simulink model "positionModeTest"  (R2022a)
settings: Solver=FixedStepAuto  StartTime=0.0  StopTime=10  FixedStep=sampleTime  RelTol=1e-3
values from neighbouring files (symbols this model uses):
  coulombTorqueNegative = theta(4)/theta(2)    [LeastSquare.m]    (also in leastSquare.m; velRide.m = resultFitNeg(2); velocityRide.m = resultFitNeg(2))
  coulombTorquePositive = theta(3)/theta(2)    [LeastSquare.m]    (also in leastSquare.m; velRide.m = resultFitPos(2); velocityRide.m = resultFitPos(2))
  inertia = 1/K_w    [LeastSquare.m]    (also in leastSquare.m)
  N = size(torqueData,1)    [coherenceTest.m]    (also in coherenceTestV2.m; fftTest.m = length(torque); firFilterParameter.m = Tout/Ts; firTest.m = Tout/Ts)
  Q0 = 0    [firFilterParameter.m]    (also in firTest.m)
  Ts = 0.001    [KalmanEstimator.m]    (also in firFilterParameter.m = samplingTime; firTest.m; leastSquare.m)
  viscousDamping = -inertia*p_w    [LeastSquare.m]    (also in leastSquare.m; velRide.m = (viscousDampingPos+viscousDampingNeg)/2; velocityRide.m = (viscousDampingPos+viscousDampingNeg)/2)
libraries: slpidlib x2
settings Model: Creator=kose  LastModifiedBy=kose
settings DataIOCC: SaveFormat=Array

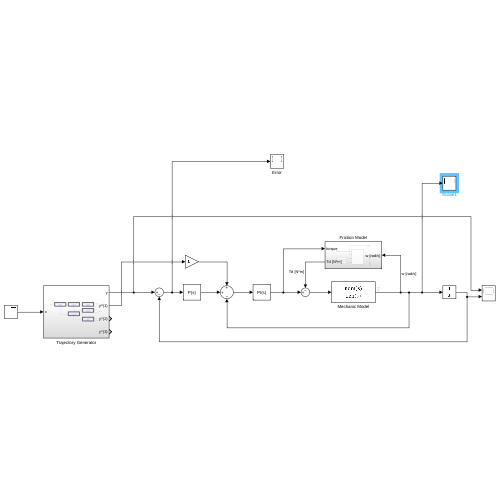
[thumbnail: Simulink's stored preview of the top-level diagram]
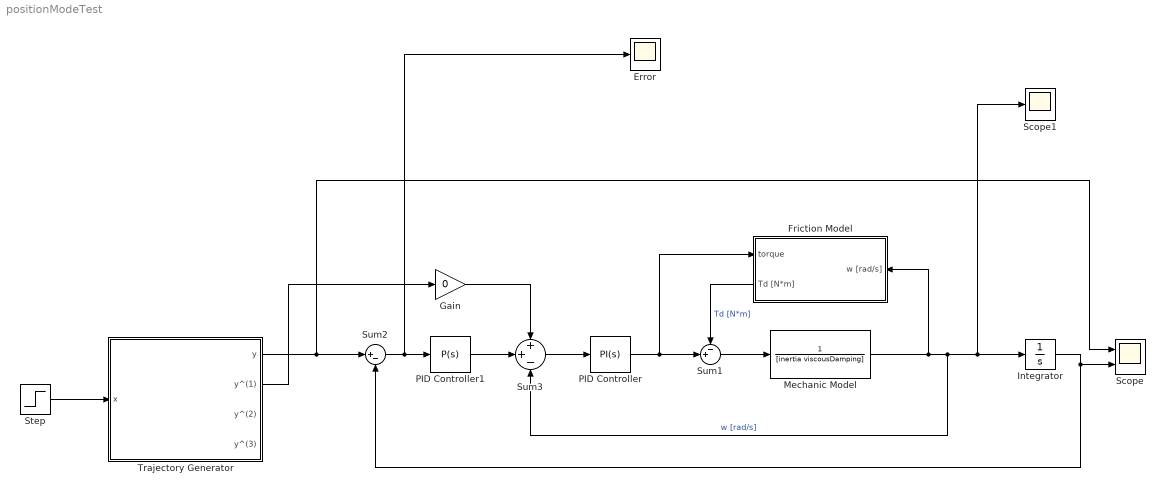
== system positionModeTest ==
  Error : Scope
  Friction Model : Subsystem
      settings: PortSchema="{\"entries\":[{\"content\":{\"sides\":[{\"content\":{\"connectorIds\":[\"In1\"]},\"type\":\"ConnectorPlacement.EquallySpacedRectSide\",\"uuid\":\"8173ecdf-76e4-4809-8dcd-ec0655641a82\"},{\"content\":{\"connectorIds\":[\"In2\",\"Out1\"],\"side\":\"RIGHT\"},\"type\":\"ConnectorPlacement.EquallySpacedRectSide\",\"uuid\":\"02bfb555-c54c-45db-8ee8-f3cb4a7ead24\"},{\"content\":{\"connectorIds\":[],\"side\":\"TOP\"},\"type\":\"ConnectorPlacement.EquallySpacedRectSide\",\"uuid\":\"776da3c7-b053-4a98-8e1b-c60377d5559b\"}]},\"type\":\"ConnectorPlacement.EquallySpacedConnector\",\"uuid\":\"773d656e-d403-490b-8d7a-ce1c081af26d\"}],\"packageUris\":[\"http://schema.mathworks.com/mf0/Connector/R2020b\"],\"version\":\"1.0\"}"
  Gain : Gain  Gain=0
  Integrator : Integrator
  Mechanic Model : TransferFcn  Denominator=[inertia viscousDamping]
  PID Controller : slpidlib/PID Controller  Controller=PI  Form=Ideal  TimeDomain=Continuous-time  UseExternalTs=off  SampleTime=-1  IntegratorMethod=Forward Euler  FilterMethod=Forward Euler  ControllerParametersSource=internal  P=1  I=1  UseKiTs=off  D=0  N=100  UseFilter=on  TunerSelectOption=Transfer Function Based (PID Tuner App)  InitialConditionSource=internal  InitialConditionForIntegrator=0  InitialConditionForFilter=0  DifferentiatorICPrevScaledInput=0  ExternalReset=none  TrackingMode=off  Kt=1  LimitOutput=off  SatLimitsSource=internal  UpperSaturationLimit=inf  LowerSaturationLimit=-inf  LinearizeAsGain=on  AntiWindupMode=none  Kb=1  POutMin=[]  POutMax=[]  IOutMin=[]  IOutMax=[]  DOutMin=[]  DOutMax=[]  NOutMin=[]  NOutMax=[]  SumOutMin=[]  SumOutMax=[]  SaturationOutMin=[]  SaturationOutMax=[]  PParamMin=[]  PParamMax=[]  IParamMin=[]  IParamMax=[]  DParamMin=[]  DParamMax=[]  NParamMin=[]  NParamMax=[]  KbParamMin=[]  KbParamMax=[]  KtParamMin=[]  KtParamMax=[]  KbOutMin=[]  KbOutMax=[]  KtOutMin=[]  KtOutMax=[]  IntegratorOutMin=[]  IntegratorOutMax=[]  FilterOutMin=[]  FilterOutMax=[]  SumI1OutMin=[]  SumI1OutMax=[]  SumI2OutMin=[]  SumI2OutMax=[]  SumI3OutMin=[]  SumI3OutMax=[]  SumI4OutMin=[]  SumI4OutMax=[]  SumDOutMin=[]  SumDOutMax=[]  DifferentiatorOutMin=[]  DifferentiatorOutMax=[]  FilterDiffOutCoefMin=[]  FilterDiffOutCoefMax=[]  ReciprocalOutMin=[]  ReciprocalOutMax=[]  SumDenOutMin=[]  SumDenOutMax=[]  SumNumOutMin=[]  SumNumOutMax=[]  DivideOutMin=[]  DivideOutMax=[]  UdiffTsProdOutMin=[]  UdiffTsProdOutMax=[]  NTsProdOutMin=[]  NTsProdOutMax=[]  UintegralTsProdOutMin=[]  UintegralTsProdOutMax=[]  UngainTsProdOutMin=[]  UngainTsProdOutMax=[]  IntegratorContinuousStateAttributes=''  IntegratorStateMustResolveToSignalObject=off  IntegratorRTWStateStorageClass=Auto  FilterContinuousStateAttributes=''  FilterStateMustResolveToSignalObject=off  FilterRTWStateStorageClass=Auto  ParallelPVariant=Passthrough  IdealPVariant=InternalParameters  IVariant=InternalParameters  DVariant=Disabled  IntegratorVariant=Continuous  SatVariant=Disabled  AWVariant=Passthrough  PCopyVariant=Disabled  TRVariant=Disabled  FdbkBlocksVariant=Forward  IdealPFdbkVariant=Disabled  SatFdbkVariant=Disabled  DerivativeFilterVariant=Disabled  NVariant=Disabled  NCopyVariant=Disabled_SignalSpec  FilterICVariant=Disabled  IntegratorICVariant=InternalICs  ExternalResetVariant=Disabled  TRSumVariant=Passthrough  SumFdbkVariant=Disabled  SumVariant=Sum_PI  TsampFilterVariant=InternalTs  TsampNgainVariant=Passthrough  TsampIntegralVariant=Passthrough  ExternalSaturationOutDataTypeStr=Inherit: Same as second input  aMode=0
  PID Controller1 : slpidlib/PID Controller  Controller=P  Form=Parallel  TimeDomain=Continuous-time  UseExternalTs=off  SampleTime=-1  IntegratorMethod=Forward Euler  FilterMethod=Forward Euler  ControllerParametersSource=internal  P=50  I=1  UseKiTs=off  D=0  N=100  UseFilter=on  TunerSelectOption=Transfer Function Based (PID Tuner App)  InitialConditionSource=internal  InitialConditionForIntegrator=0  InitialConditionForFilter=0  DifferentiatorICPrevScaledInput=0  ExternalReset=none  TrackingMode=off  Kt=1  LimitOutput=off  SatLimitsSource=internal  UpperSaturationLimit=inf  LowerSaturationLimit=-inf  LinearizeAsGain=on  AntiWindupMode=none  Kb=1  POutMin=[]  POutMax=[]  IOutMin=[]  IOutMax=[]  DOutMin=[]  DOutMax=[]  NOutMin=[]  NOutMax=[]  SumOutMin=[]  SumOutMax=[]  SaturationOutMin=[]  SaturationOutMax=[]  PParamMin=[]  PParamMax=[]  IParamMin=[]  IParamMax=[]  DParamMin=[]  DParamMax=[]  NParamMin=[]  NParamMax=[]  KbParamMin=[]  KbParamMax=[]  KtParamMin=[]  KtParamMax=[]  KbOutMin=[]  KbOutMax=[]  KtOutMin=[]  KtOutMax=[]  IntegratorOutMin=[]  IntegratorOutMax=[]  FilterOutMin=[]  FilterOutMax=[]  SumI1OutMin=[]  SumI1OutMax=[]  SumI2OutMin=[]  SumI2OutMax=[]  SumI3OutMin=[]  SumI3OutMax=[]  SumI4OutMin=[]  SumI4OutMax=[]  SumDOutMin=[]  SumDOutMax=[]  DifferentiatorOutMin=[]  DifferentiatorOutMax=[]  FilterDiffOutCoefMin=[]  FilterDiffOutCoefMax=[]  ReciprocalOutMin=[]  ReciprocalOutMax=[]  SumDenOutMin=[]  SumDenOutMax=[]  SumNumOutMin=[]  SumNumOutMax=[]  DivideOutMin=[]  DivideOutMax=[]  UdiffTsProdOutMin=[]  UdiffTsProdOutMax=[]  NTsProdOutMin=[]  NTsProdOutMax=[]  UintegralTsProdOutMin=[]  UintegralTsProdOutMax=[]  UngainTsProdOutMin=[]  UngainTsProdOutMax=[]  IntegratorContinuousStateAttributes=''  IntegratorStateMustResolveToSignalObject=off  IntegratorRTWStateStorageClass=Auto  FilterContinuousStateAttributes=''  FilterStateMustResolveToSignalObject=off  FilterRTWStateStorageClass=Auto  ParallelPVariant=InternalParameters  IdealPVariant=Disabled  IVariant=Disabled  DVariant=Disabled  IntegratorVariant=Disabled  SatVariant=Disabled  AWVariant=Disabled  PCopyVariant=Disabled  TRVariant=Disabled  FdbkBlocksVariant=Forward  IdealPFdbkVariant=Disabled  SatFdbkVariant=Disabled  DerivativeFilterVariant=Disabled  NVariant=Disabled  NCopyVariant=Disabled_SignalSpec  FilterICVariant=Disabled  IntegratorICVariant=Disabled  ExternalResetVariant=Disabled  TRSumVariant=Passthrough  SumFdbkVariant=Disabled  SumVariant=Passthrough_P  TsampFilterVariant=InternalTs  TsampNgainVariant=Passthrough  TsampIntegralVariant=Disabled_SignalSpec  ExternalSaturationOutDataTypeStr=Inherit: Same as second input  aMode=0
  Scope : Scope  NumInputPorts=2
  Scope1 : Scope
  Step : Step  Time=0  After=100  SampleTime=0.001
  Sum1 : Sum  Inputs=-+|
  Sum2 : Sum  Inputs=|+-
  Sum3 : Sum  Inputs=++-
  Trajectory Generator : Subsystem
  wires:
  Mechanic Model/1 -> Sum3/3, Scope1/1, Integrator/1, Friction Model/1(w [rad/s])  "w [rad/s]"
  Sum1/1 -> Mechanic Model/1
  Friction Model/1(Td [N*m]) -> Sum1/1  "Td [N*m]"
  PID Controller/1 -> Friction Model/2(torque), Sum1/2
  Sum2/1 -> Error/1, PID Controller1/1
  Integrator/1 -> Scope/2, Sum2/2
  Step/1 -> Trajectory Generator/1(x)
  Trajectory Generator/1(y) -> Scope/1, Sum2/1
  Sum3/1 -> PID Controller/1
  PID Controller1/1 -> Sum3/2
  Trajectory Generator/2(y^(1)) -> Gain/1
  Gain/1 -> Sum3/1

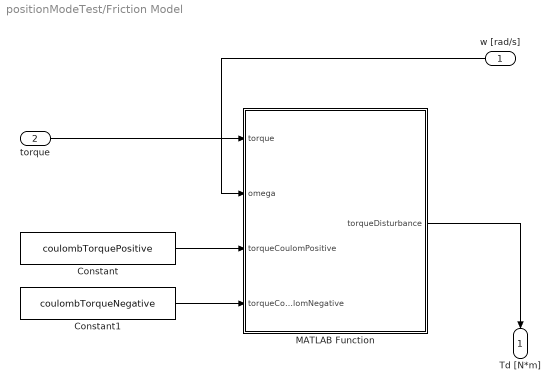
== system positionModeTest/Friction Model ==
  w [rad/s] : Inport
  torque : Inport  Port=2
  Constant : Constant  Value=coulombTorquePositive
  Constant1 : Constant  Value=coulombTorqueNegative
  MATLAB Function : MATLAB Function  TreatAsAtomicUnit=on
  Td [N*m] : Outport
  wires:
  w [rad/s]/1 -> MATLAB Function/2(omega)
  Constant/1 -> MATLAB Function/3(torqueCoulomPositive)
  torque/1 -> MATLAB Function/1(torque)
  MATLAB Function/1(torqueDisturbance) -> Td [N*m]/1
  Constant1/1 -> MATLAB Function/4(torqueCoulomNegative)

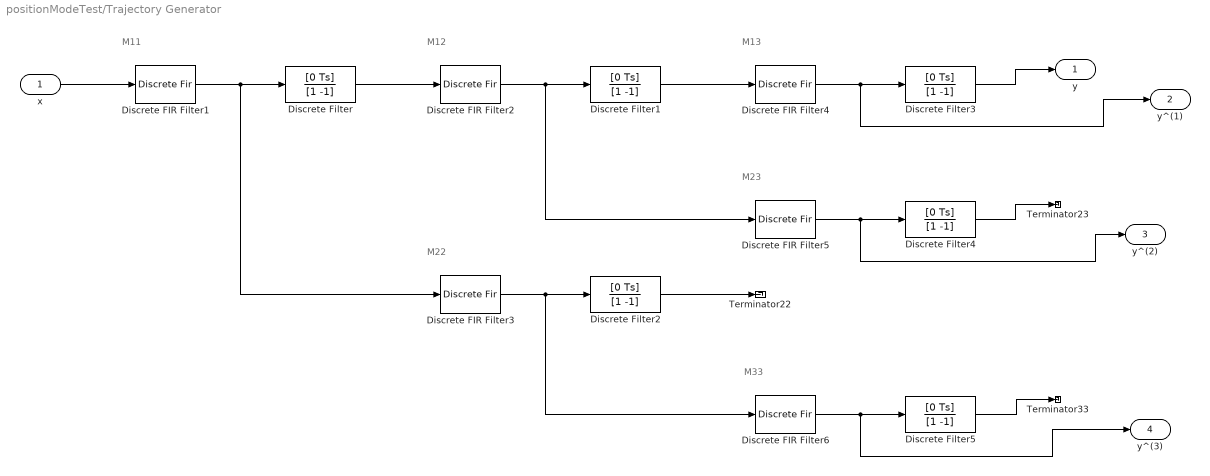
== system positionModeTest/Trajectory Generator ==
  note: M33
  note: M23
  note: M13
  note: M22
  note: M12
  note: M11
  x : Inport
  Discrete FIR Filter1 : DiscreteFir  Coefficients=1/N(1)/Ts*[1 zeros(1,N(1)-1) -1]  InitialStates=Q0  SampleTime=Ts
  Discrete FIR Filter2 : DiscreteFir  Coefficients=1/N(2)/Ts*[1 zeros(1,N(2)-1) -1]  InitialStates=Q0  SampleTime=Ts
  Discrete FIR Filter3 : DiscreteFir  Coefficients=1/N(2)/Ts*[1 zeros(1,N(2)-1) -1]  InitialStates=Q0  SampleTime=Ts
  Discrete FIR Filter4 : DiscreteFir  Coefficients=1/N(3)/Ts*[1 zeros(1,N(3)-1) -1]  InitialStates=Q0  SampleTime=Ts
  Discrete FIR Filter5 : DiscreteFir  Coefficients=1/N(3)/Ts*[1 zeros(1,N(3)-1) -1]  InitialStates=Q0  SampleTime=Ts
  Discrete FIR Filter6 : DiscreteFir  Coefficients=1/N(3)/Ts*[1 zeros(1,N(3)-1) -1]  InitialStates=Q0  SampleTime=Ts
  Discrete Filter{,1..5} (6 alike) : DiscreteFilter  Numerator=[0 Ts]  Denominator=[1 -1]  InitialStates=Q0  SampleTime=Ts
  Terminator22 : Terminator
  Terminator23 : Terminator
  Terminator33 : Terminator
  y : Outport
  y^(1) : Outport  Port=2
  y^(2) : Outport  Port=3
  y^(3) : Outport  Port=4
  wires:
  Discrete Filter2/1 -> Terminator22/1
  Discrete Filter4/1 -> Terminator23/1
  Discrete Filter5/1 -> Terminator33/1
  Discrete Filter3/1 -> y/1
  Discrete FIR Filter4/1 -> y^(1)/1, Discrete Filter3/1
  Discrete FIR Filter5/1 -> y^(2)/1, Discrete Filter4/1
  Discrete FIR Filter6/1 -> y^(3)/1, Discrete Filter5/1
  x/1 -> Discrete FIR Filter1/1
  Discrete Filter/1 -> Discrete FIR Filter2/1
  Discrete FIR Filter1/1 -> Discrete FIR Filter3/1, Discrete Filter/1
  Discrete Filter1/1 -> Discrete FIR Filter4/1
  Discrete FIR Filter2/1 -> Discrete FIR Filter5/1, Discrete Filter1/1
  Discrete FIR Filter3/1 -> Discrete FIR Filter6/1, Discrete Filter2/1

== matlab function positionModeTest/Friction Model/MATLAB Function ==
  data: torque input; torqueDisturbance output; omega input; torqueCoulomPositive input; torqueCoulomNegative input
function torqueDisturbance = fcn(torque, omega, torqueCoulomPositive, torqueCoulomNegative)

if omega > 0
    torqueDisturbance = torqueCoulomPositive;
elseif omega < 0
    torqueDisturbance = torqueCoulomNegative;    
elseif omega == 0 &&  torque < torqueCoulomPositive
    torqueDisturbance = torque;
elseif omega == 0 && torque < torqueCoulomNegative
    torqueDisturbance = torque;
else
    torqueDisturbance = 0;
end
end
